simulink model "Senorless"  (R2023a)
settings: Solver=FixedStepDiscrete  StartTime=0.0  StopTime=5  FixedStep=1/FOC_FRQ  RelTol=1e-3
values from neighbouring files (symbols this model uses):
  ADC_REF = 3.6    [Senorless.sldd]
  ADC_SAMPLE_MAX = 32767.0    [Senorless.sldd]
  AMP_GAIN = 16.0    [Senorless.sldd]
  CURR_INPUT = 3276.0    [Senorless.sldd]
  CURR_KI = 380.0    [Senorless.sldd]
  CURR_KP = 0.04    [Senorless.sldd]
  CURR_LIMIT = 0.95    [Senorless.sldd]
  CURR_OVER = 6.0    [Senorless.sldd]
  CURR_POINT_GAIN = 7.0    [Senorless.sldd]
  CURR_STEP = 32760.0    [Senorless.sldd]
  CURR_UNDER = 0.03    [Senorless.sldd]
  CURR_WIDTH = 6552.0    [Senorless.sldd]
  FOC_FRQ = 25000.0    [Senorless.sldd]
  GAMMA = 32767.0    [Senorless.sldd]
  IMAX = 10.0    [Senorless.sldd]
  LPF_FRQ = 2000.0    [Senorless.sldd]
  MOTOR_DAMPER = 2.06E-7    [Senorless.sldd]
  MOTOR_FLUX = 0.00212352    [Senorless.sldd]
  MOTOR_INERTIA = 4.0E-7    [Senorless.sldd]
  MOTOR_LS = 0.000536    [Senorless.sldd]
  MOTOR_PN = 7.0    [Senorless.sldd]
  MOTOR_RS = 4.0    [Senorless.sldd]
  OPEN_IQ = 0.28    [Senorless.sldd]
  OPEN_IQ_MIN = 0.05    [Senorless.sldd]
  OPEN_IQ_SLOW = 0.1    [Senorless.sldd]
  OPEN_SPD = 1000.0    [Senorless.sldd]
  OPEN_SPD_SLOW = 180.0    [Senorless.sldd]
  OPEN_TIME = 0.5    [Senorless.sldd]
  OPEN_TIME_NFO = 0.5    [Senorless.sldd]
  PLL_LIMIT = 0.9    [Senorless.sldd]
  PLL_WIDTH = 800.0    [Senorless.sldd]
  PWM_FRQ = 96000000.0    [Senorless.sldd]
  RS_HUNT = 0.02    [Senorless.sldd]
  SMOK_FRQ = 600.0    [Senorless.sldd]
  SPD_LIMIT = 0.9    [Senorless.sldd]
  SPD_LPF_LEVEL = 0.0    [Senorless.sldd]
  SPD_MAX = 12000.0    [Senorless.sldd]
  SPD_MIN = 4000.0    [Senorless.sldd]
  SPD_REDUCE = 380.0    [Senorless.sldd]
  SPD_STEP = 6.0    [Senorless.sldd]
  SPD_WIDTH = 20.0    [Senorless.sldd]
  THETA_ERR_LIMIT = 8192.0    [Senorless.sldd]
  TS_POINT_GAIN = 10.0    [Senorless.sldd]
  UDC = 48.0    [Senorless.sldd]
  UDC_GAIN = 21.0    [Senorless.sldd]
  UDC_POINT_GAIN = 10.0    [Senorless.sldd]
undefined symbols (not defined in the file or in its folder): curr_q_ki, curr_q_kp, DiscIntNeverNeededParam, magnitude, PLL_LPF_LEVEL, Udc
libraries: simulink x20, slpidlib x5, mcbcontrolslib x2, mcbplantlib x1, autolibpmsmexterior x1, spspowerguiLib x1
(part 7 of 8)

== system Senorless/FOC_PointModel/idq_Controller/PI Controller2/积分器//双边沿初始化 ==
  Ki : Inport
  input : Inport  Port=2
  Xo : Inport  Port=3
  Reset : Inport  Port=4
  Constant : Constant  Value=32767*32767  OutDataTypeStr=int32
  Data Store Memory : DataStoreMemory  DataStoreName=tmp  WriteAfterWriteMsg=warning  ShowAdditionalParam=off  OutDataTypeStr=int32
  Data Store Read : DataStoreRead  DataStoreName=tmp  IndexOptions=Index vector (dialog)  Indices=1  OutputSizes=1
  Data Store Read1 : DataStoreRead  DataStoreName=Ts_Point  IndexOptions=Index vector (dialog)  Indices=1  OutputSizes=1
  Data Store Read3 : DataStoreRead  DataStoreName=Curr_Limit  IndexOptions=Index vector (dialog)  Indices=1  OutputSizes=1
  Data Store Write : DataStoreWrite  DataStoreName=tmp  IndexOptions=Index vector (dialog)  Indices=1  OutputSizes=1
  Data Type Conversion : DataTypeConversion  OutDataTypeStr=int16  SaturateOnIntegerOverflow=off
  Data Type Conversion2 : DataTypeConversion  OutDataTypeStr=int32  SaturateOnIntegerOverflow=off
  Data Type Conversion3 : DataTypeConversion  Commented=on  OutDataTypeStr=int16  SaturateOnIntegerOverflow=off
  Divide : Product  Commented=on  Inputs=*/  OutDataTypeStr=int32  RndMeth=Zero
  Gain : Gain  Gain=-1  OutDataTypeStr=int32  RndMeth=Zero
  Gain1 : Gain  Gain=-1  OutDataTypeStr=int32  RndMeth=Zero
  MATLAB Function : MATLAB Function  TreatAsAtomicUnit=on
  MATLAB Function1 : MATLAB Function  TreatAsAtomicUnit=on
  MATLAB Function2 : MATLAB Function  TreatAsAtomicUnit=on
  Product1 : Product  OutDataTypeStr=int32  RndMeth=Zero
  Product2 : Product  OutDataTypeStr=int32  RndMeth=Zero
  Reset_Block : Subsystem
  Scope : Scope  NumInputPorts=2
  Sum : Sum  Inputs=|++  OutDataTypeStr=int32  RndMeth=Zero
  Sum1 : Sum  Inputs=|+-  OutDataTypeStr=int32  RndMeth=Zero
  Sum2 : Sum  Inputs=-+  OutDataTypeStr=int32  RndMeth=Zero
  Ts适当放大的缩小系数， 详见初始化模块 : ArithShift  Commented=on  BitShiftNumber=TS_POINT_GAIN  DiagnosticForOORShift=Error
  Unit Delay : UnitDelay  SampleTime=-1  HasFrameUpgradeWarning=on
  周期定点化适当放大2^n : Constant  Value=TS_POINT_GAIN
  积分器运行频率 : Constant  Commented=on  Value=FOC_FRQ
  这个是缩小周期增益的 : ArithShift  BitShiftNumber=15  DiagnosticForOORShift=Error
  output : Outport
  wires:
  Data Type Conversion/1 -> Product1/2
  MATLAB Function1/1(out) -> Sum/1, Sum1/2, Scope/2
  [Limit1] -> MATLAB Function1/2(up), Gain1/1
  Gain1/1 -> MATLAB Function1/3(low)
  [limit] -> MATLAB Function/2(up), Gain/1
  Gain/1 -> MATLAB Function/3(low)
  Sum2/1 -> [Limit1]
  Data Store Read3/1 -> [limit], Sum2/1
  Constant/1 -> Sum2/2
  周期定点化适当放大2^n/1 -> MATLAB Function2/2(n)
  input/1 -> Product2/2
  Data Store Read1/1 -> Product2/1
  Sum1/1 -> Reset_Block/1(Xo)
  Data Type Conversion2/1 -> Sum1/1
  Product1/1 -> MATLAB Function1/1(in), Scope/1
  Sum/1 -> MATLAB Function/1(in)
  MATLAB Function2/1(out) -> Product1/1
  Reset/1 -> Reset_Block/Trigger
  Ki/1 -> MATLAB Function2/1(in)
  这个是缩小周期增益的/1 -> Data Type Conversion/1
  Product2/1 -> 这个是缩小周期增益的/1
  Data Type Conversion3/1 -> Divide/2
  Xo/1 -> Data Type Conversion2/1
  积分器运行频率/1 -> Data Type Conversion3/1
  Unit Delay/1 -> Data Store Write/1
  Data Store Read/1 -> Sum/2
  MATLAB Function/1(out) -> Unit Delay/1, output/1

== system Senorless/FOC_PointModel/加速强拖/加速积分角度/积分器 ==
  K_p : Inport
  input : Inport  Port=2
  Xo : Inport  Port=3
  Reset : Inport  Port=4
  Data Store Memory : DataStoreMemory  DataStoreName=tmp  WriteAfterWriteMsg=warning  ShowAdditionalParam=off
  Data Store Read : DataStoreRead  DataStoreName=tmp  IndexOptions=Index vector (dialog)  Indices=1  OutputSizes=1
  Data Store Write : DataStoreWrite  DataStoreName=tmp  IndexOptions=Index vector (dialog)  Indices=1  OutputSizes=1
  Data Type Conversion2 : DataTypeConversion  OutDataTypeStr=int32  SaturateOnIntegerOverflow=off
  Data Type Conversion3 : DataTypeConversion  OutDataTypeStr=int32  SaturateOnIntegerOverflow=off
  Divide : Product  Inputs=*/  OutDataTypeStr=int32  RndMeth=Zero
  Product : Product  OutDataTypeStr=int64  RndMeth=Zero
  Product1 : Product  OutDataTypeStr=int64  RndMeth=Zero
  Reset_Block : Subsystem
  Sum : Sum  Inputs=|++  OutDataTypeStr=int64  RndMeth=Zero
  Unit Delay : UnitDelay  SampleTime=-1  HasFrameUpgradeWarning=on
  积分器运行频率 : Constant  Value=FOC_FRQ
  output : Outport
  wires:
  K_p/1 -> Product1/1, Product/2
  Reset/1 -> Reset_Block/Trigger
  Data Store Read/1 -> Sum/2
  Unit Delay/1 -> Data Store Write/1
  Product/1 -> Reset_Block/1(Xo)
  Divide/1 -> Product1/2
  input/1 -> Divide/1
  Product1/1 -> Sum/1
  积分器运行频率/1 -> Data Type Conversion3/1
  Data Type Conversion3/1 -> Divide/2
  Xo/1 -> Data Type Conversion2/1
  Data Type Conversion2/1 -> Product/1
  Sum/1 -> Unit Delay/1, output/1

== system Senorless/FOC_PointModel/加速强拖/加速积分角度/积分器2 ==
  note: 此处相减作用是与后面的++相抵消，这样初始化后第一个输出值就是reset值，不然是reset值+Kp*input值
  K_p : Inport
  input : Inport  Port=2
  Xo : Inport  Port=3
  Reset : Inport  Port=4
  Data Store Memory : DataStoreMemory  DataStoreName=tmp  WriteAfterWriteMsg=warning  ShowAdditionalParam=off
  Data Store Read : DataStoreRead  DataStoreName=tmp  IndexOptions=Index vector (dialog)  Indices=1  OutputSizes=1
  Data Store Write : DataStoreWrite  DataStoreName=tmp  IndexOptions=Index vector (dialog)  Indices=1  OutputSizes=1
  Data Type Conversion2 : DataTypeConversion  OutDataTypeStr=int32  SaturateOnIntegerOverflow=off
  Data Type Conversion3 : DataTypeConversion  OutDataTypeStr=int32  SaturateOnIntegerOverflow=off
  Divide : Product  Inputs=*/  OutDataTypeStr=int32  RndMeth=Zero
  Product : Product  OutDataTypeStr=int64  RndMeth=Zero
  Product1 : Product  OutDataTypeStr=int64  RndMeth=Zero
  Reset_Block : Subsystem
  Sum : Sum  Inputs=|++  OutDataTypeStr=int64  RndMeth=Zero
  Sum1 : Sum  Inputs=|+-  OutDataTypeStr=int64  RndMeth=Zero
  Unit Delay : UnitDelay  SampleTime=-1  HasFrameUpgradeWarning=on
  积分器运行频率 : Constant  Value=FOC_FRQ
  output : Outport
  wires:
  K_p/1 -> Product1/1, Product/2
  Reset/1 -> Reset_Block/Trigger
  Data Store Read/1 -> Sum/2
  Sum/1 -> Unit Delay/1, output/1
  Unit Delay/1 -> Data Store Write/1
  Product/1 -> Sum1/1
  Divide/1 -> Product1/2
  input/1 -> Divide/1
  Product1/1 -> Sum1/2, Sum/1
  积分器运行频率/1 -> Data Type Conversion3/1
  Data Type Conversion3/1 -> Divide/2
  Xo/1 -> Data Type Conversion2/1
  Data Type Conversion2/1 -> Product/1
  Sum1/1 -> Reset_Block/1(Xo)

== system Senorless/FOC_PointModel/加速强拖/加速积分角度/积分器3 ==
  input : Inport
  Constant : Constant  OutDataTypeStr=int16
  Data Store Read1 : DataStoreRead  DataStoreName=Ts_Point  IndexOptions=Index vector (dialog)  Indices=1  OutputSizes=1
  Product1 : Product  OutDataTypeStr=int32  RndMeth=Zero
  Product2 : Product  OutDataTypeStr=int32  RndMeth=Zero
  Shift Arithmetic : ArithShift  BitShiftNumberSource=Input port  BitShiftNumber=8  BitShiftDirection=Right
      settings: InputPortMap=u0,p1
  Sum : Sum  Inputs=++|  OutDataTypeStr=int32  RndMeth=Zero
  Unit Delay : UnitDelay  SampleTime=-1  HasFrameUpgradeWarning=on
  周期定点化适当放大2^n : Constant  Value=TS_POINT_GAIN
  这个是缩小周期增益的 : ArithShift  BitShiftNumber=15  DiagnosticForOORShift=Error
  output : Outport
  wires:
  周期定点化适当放大2^n/1 -> Shift Arithmetic/2
  Shift Arithmetic/1 -> Product2/2
  Data Store Read1/1 -> Product2/1
  input/1 -> Shift Arithmetic/1
  Product2/1 -> 这个是缩小周期增益的/1
  Sum/1 -> Unit Delay/1, output/1
  这个是缩小周期增益的/1 -> Product1/1
  Constant/1 -> Product1/2
  Product1/1 -> Sum/2
  Unit Delay/1 -> Sum/1

== system Senorless/FOC_PointModel/加速强拖/加速积分角度/积分器4 ==
  input : Inport
  Constant : Constant  OutDataTypeStr=int16
  Data Store Read1 : DataStoreRead  DataStoreName=Ts_Point  IndexOptions=Index vector (dialog)  Indices=1  OutputSizes=1
  Product1 : Product  OutDataTypeStr=int32  RndMeth=Zero
  Product2 : Product  OutDataTypeStr=int32  RndMeth=Zero
  Shift Arithmetic : ArithShift  BitShiftNumberSource=Input port  BitShiftNumber=8  BitShiftDirection=Right
      settings: InputPortMap=u0,p1
  Sum : Sum  Inputs=++|  OutDataTypeStr=int32  RndMeth=Zero
  Unit Delay : UnitDelay  SampleTime=-1  HasFrameUpgradeWarning=on
  周期定点化适当放大2^n : Constant  Value=TS_POINT_GAIN
  这个是缩小周期增益的 : ArithShift  BitShiftNumber=15  DiagnosticForOORShift=Error
  output : Outport
  wires:
  Unit Delay/1 -> Sum/1
  Product1/1 -> Sum/2
  Constant/1 -> Product1/2
  这个是缩小周期增益的/1 -> Product1/1
  Sum/1 -> output/1, Unit Delay/1
  Product2/1 -> 这个是缩小周期增益的/1
  input/1 -> Shift Arithmetic/1
  Data Store Read1/1 -> Product2/1
  Shift Arithmetic/1 -> Product2/2
  周期定点化适当放大2^n/1 -> Shift Arithmetic/2

== system Senorless/FOC_PointModel/观测器闭环//速度环/PI Controller/积分器 ==
  Ki : Inport
  input : Inport  Port=2
  Constant : Constant  Value=32767  OutDataTypeStr=int32
  Data Store Read1 : DataStoreRead  DataStoreName=Ts_Point  IndexOptions=Index vector (dialog)  Indices=1  OutputSizes=1
  Data Store Read3 : DataStoreRead  DataStoreName=Speed_Limit  IndexOptions=Index vector (dialog)  Indices=1  OutputSizes=1
  Data Type Conversion1 : DataTypeConversion  OutDataTypeStr=int16  SaturateOnIntegerOverflow=off
  Gain1 : Gain  Gain=-1  OutDataTypeStr=int32  RndMeth=Zero
  Gain2 : Gain  Gain=-1  OutDataTypeStr=int32  RndMeth=Zero
  MATLAB Function : MATLAB Function  TreatAsAtomicUnit=on
  MATLAB Function1 : MATLAB Function  TreatAsAtomicUnit=on
  Product1 : Product  OutDataTypeStr=int32  RndMeth=Zero
  Product2 : Product  OutDataTypeStr=int32  RndMeth=Zero
  Scope : Scope  NumInputPorts=2
  Shift Arithmetic : ArithShift  BitShiftNumberSource=Input port  BitShiftNumber=8  BitShiftDirection=Right
      settings: InputPortMap=u0,p1
  Sum : Sum  Inputs=|++  OutDataTypeStr=int32  RndMeth=Zero
  Sum2 : Sum  Inputs=-+  OutDataTypeStr=int32  RndMeth=Zero
  Unit Delay : UnitDelay  SampleTime=-1  HasFrameUpgradeWarning=on
  周期定点化适当放大2^n : Constant  Value=TS_POINT_GAIN
  这个是缩小周期增益的 : ArithShift  BitShiftNumber=15  DiagnosticForOORShift=Warning
  output : Outport
  wires:
  Constant/1 -> Sum2/2
  Sum2/1 -> [Limit1]
  [limit] -> Gain2/1, MATLAB Function/2(up)
  Gain1/1 -> MATLAB Function1/3(low)
  [Limit1] -> Gain1/1, MATLAB Function1/2(up)
  MATLAB Function1/1(out) -> Sum/1
  Sum/1 -> MATLAB Function/1(in)
  Ki/1 -> Product1/1
  Product2/1 -> Shift Arithmetic/1
  Data Store Read1/1 -> Product2/1
  周期定点化适当放大2^n/1 -> Shift Arithmetic/2
  MATLAB Function/1(out) -> Unit Delay/1, output/1
  input/1 -> Product2/2
  Product1/1 -> 这个是缩小周期增益的/1
  这个是缩小周期增益的/1 -> MATLAB Function1/1(in)
  Data Store Read3/1 -> Sum2/1, [limit]
  Data Type Conversion1/1 -> Scope/1, Product1/2
  Gain2/1 -> MATLAB Function/3(low)
  Shift Arithmetic/1 -> Scope/2, Data Type Conversion1/1
  Unit Delay/1 -> Sum/2

== system Senorless/FOC_PointModel/观测器闭环//速度环/积分器//上升沿初始化/Reset_Block ==
  Xo : Inport
  Trigger : TriggerPort  VariantControl=(inherit)  OutputDataType=int8  InitialTriggerSignalState=zero  PortDimensions=1
  Data Store Write1 : DataStoreWrite  DataStoreName=tmp  IndexOptions=Index vector (dialog)  Indices=1  OutputSizes=1
  wires:
  Xo/1 -> Data Store Write1/1

== system Senorless/FOC_PointModel/Observers/PLL/PI Controller/积分器 ==
  Ki : Inport
  input : Inport  Port=2
  Constant : Constant  Value=32767*32767  OutDataTypeStr=int32
  Data Store Read1 : DataStoreRead  DataStoreName=Ts_Point  IndexOptions=Index vector (dialog)  Indices=1  OutputSizes=1
  Data Store Read3 : DataStoreRead  DataStoreName=PLL_Limit  IndexOptions=Index vector (dialog)  Indices=1  OutputSizes=1
  Data Type Conversion3 : DataTypeConversion  Commented=on  OutDataTypeStr=int16  SaturateOnIntegerOverflow=off
  Divide : Product  Commented=on  Inputs=*/  OutDataTypeStr=int32  RndMeth=Zero
  Gain : Gain  Gain=-1  OutDataTypeStr=int32  RndMeth=Zero
  Product1 : Product  OutDataTypeStr=int32  RndMeth=Zero
  Product2 : Product  OutDataTypeStr=int32  RndMeth=Zero
  Saturation Dynamic2 : simulink/Discontinuities/Saturation Dynamic  OutMin=[]  OutMax=[]  OutDataTypeStr=Inherit: Same as second input  OutDataType=fixdt(1, 16)  OutScaling=2^-10  RndMeth=Zero  DoSatur=off
  Shift Arithmetic : ArithShift  BitShiftNumberSource=Input port  BitShiftNumber=8  BitShiftDirection=Right
      settings: InputPortMap=u0,p1
  Sum : Sum  Inputs=|++  OutDataTypeStr=int32  RndMeth=Zero
  Sum2 : Sum  Inputs=-+  OutDataTypeStr=int32  RndMeth=Zero
  Ts适当放大的缩小系数， 详见初始化模块 : ArithShift  Commented=on  BitShiftNumber=TS_POINT_GAIN  DiagnosticForOORShift=Error
  Unit Delay : UnitDelay  SampleTime=-1  HasFrameUpgradeWarning=on
  周期定点化适当放大2^n : Constant  Value=TS_POINT_GAIN
  积分器运行频率 : Constant  Commented=on  Value=FOC_FRQ
  这个是缩小周期增益的 : ArithShift  BitShiftNumber=15  DiagnosticForOORShift=Error
  output : Outport
  wires:
  积分器运行频率/1 -> Data Type Conversion3/1
  Data Type Conversion3/1 -> Divide/2
  Product2/1 -> 这个是缩小周期增益的/1
  Ki/1 -> Shift Arithmetic/1
  Shift Arithmetic/1 -> Product1/1
  Data Store Read1/1 -> Product2/1
  input/1 -> Product2/2
  周期定点化适当放大2^n/1 -> Shift Arithmetic/2
  [Limit] -> Gain/1
  Data Store Read3/1 -> Sum2/1, [Limit]
  Constant/1 -> Sum2/2
  Sum2/1 -> [Limit1]
  这个是缩小周期增益的/1 -> Product1/2
  Unit Delay/1 -> Sum/2
  Gain/1 -> Saturation Dynamic2/3
  Sum/1 -> Saturation Dynamic2/2
  [Limit] -> Saturation Dynamic2/1
  Saturation Dynamic2/1 -> Unit Delay/1, output/1
  Product1/1 -> Sum/1

== system Senorless/FOC_PointModel/Observers/PLL2/PI Controller/积分器 ==
  Ki : Inport
  input : Inport  Port=2
  Constant : Constant  Value=32767*32767  OutDataTypeStr=int32
  Data Store Read1 : DataStoreRead  DataStoreName=Ts_Point  IndexOptions=Index vector (dialog)  Indices=1  OutputSizes=1
  Data Store Read3 : DataStoreRead  DataStoreName=PLL_Limit  IndexOptions=Index vector (dialog)  Indices=1  OutputSizes=1
  Data Type Conversion3 : DataTypeConversion  Commented=on  OutDataTypeStr=int16  SaturateOnIntegerOverflow=off
  Divide : Product  Commented=on  Inputs=*/  OutDataTypeStr=int32  RndMeth=Zero
  Gain : Gain  Gain=-1  OutDataTypeStr=int32  RndMeth=Zero
  Product1 : Product  OutDataTypeStr=int32  RndMeth=Zero
  Product2 : Product  OutDataTypeStr=int32  RndMeth=Zero
  Saturation Dynamic2 : simulink/Discontinuities/Saturation Dynamic  OutMin=[]  OutMax=[]  OutDataTypeStr=Inherit: Same as second input  OutDataType=fixdt(1, 16)  OutScaling=2^-10  RndMeth=Zero  DoSatur=off
  Shift Arithmetic : ArithShift  BitShiftNumberSource=Input port  BitShiftNumber=8  BitShiftDirection=Right
      settings: InputPortMap=u0,p1
  Sum : Sum  Inputs=|++  OutDataTypeStr=int32  RndMeth=Zero
  Sum2 : Sum  Inputs=-+  OutDataTypeStr=int32  RndMeth=Zero
  Ts适当放大的缩小系数， 详见初始化模块 : ArithShift  Commented=on  BitShiftNumber=TS_POINT_GAIN  DiagnosticForOORShift=Error
  Unit Delay : UnitDelay  SampleTime=-1  HasFrameUpgradeWarning=on
  周期定点化适当放大2^n : Constant  Value=TS_POINT_GAIN
  积分器运行频率 : Constant  Commented=on  Value=FOC_FRQ
  这个是缩小周期增益的 : ArithShift  BitShiftNumber=15  DiagnosticForOORShift=Error
  output : Outport
  wires:
  Product1/1 -> Sum/1
  Saturation Dynamic2/1 -> output/1, Unit Delay/1
  [Limit] -> Saturation Dynamic2/1
  Sum/1 -> Saturation Dynamic2/2
  Gain/1 -> Saturation Dynamic2/3
  Unit Delay/1 -> Sum/2
  这个是缩小周期增益的/1 -> Product1/2
  Sum2/1 -> [Limit1]
  Constant/1 -> Sum2/2
  Data Store Read3/1 -> [Limit], Sum2/1
  [Limit] -> Gain/1
  周期定点化适当放大2^n/1 -> Shift Arithmetic/2
  input/1 -> Product2/2
  Data Store Read1/1 -> Product2/1
  Shift Arithmetic/1 -> Product1/1
  Ki/1 -> Shift Arithmetic/1
  Product2/1 -> 这个是缩小周期增益的/1
  Data Type Conversion3/1 -> Divide/2
  积分器运行频率/1 -> Data Type Conversion3/1

== system Senorless/FOC_PointModel/idq_Controller/PI Controller2/积分器//双边沿初始化/Reset_Block ==
  Xo : Inport
  Trigger : TriggerPort  TriggerType=either  VariantControl=(inherit)  OutputDataType=int8  InitialTriggerSignalState=zero  PortDimensions=1
  Data Store Write1 : DataStoreWrite  DataStoreName=tmp  IndexOptions=Index vector (dialog)  Indices=1  OutputSizes=1
  wires:
  Xo/1 -> Data Store Write1/1

== system Senorless/FOC_PointModel/加速强拖/加速积分角度/积分器/Reset_Block ==
  Xo : Inport
  Trigger : TriggerPort  VariantControl=(inherit)  OutputDataType=int8  InitialTriggerSignalState=zero  PortDimensions=1
  Data Store Write1 : DataStoreWrite  DataStoreName=tmp  IndexOptions=Index vector (dialog)  Indices=1  OutputSizes=1
  wires:
  Xo/1 -> Data Store Write1/1

== system Senorless/FOC_PointModel/加速强拖/加速积分角度/积分器2/Reset_Block ==
  Xo : Inport
  Trigger : TriggerPort  VariantControl=(inherit)  OutputDataType=int8  InitialTriggerSignalState=zero  PortDimensions=1
  Data Store Write1 : DataStoreWrite  DataStoreName=tmp  IndexOptions=Index vector (dialog)  Indices=1  OutputSizes=1
  wires:
  Xo/1 -> Data Store Write1/1

== stateflow chart Senorless/FOC_PointModel/Chart ==
  state StopStage%出错暂停
    en:
    du:
    Reset = 1;
    ex:
  state IDLE
    en:
    du:
    Motor_State = 0;
    Reset = 0;
    ex:
  state SlowOpen%缓慢强拖
    en:
    du:
    Motor_State = 5;
    Reset = 0;
    ex:
  state AlignStage%对齐
    en:
    du:
    Motor_State = 1;
    ex:
  state OpenStage%降力矩
    en:
    Over_Curr_Cnt = 0;
    du:
    Motor_State = 3;
    ex:
  state SpeedupStage%加速
    en:
    du:
    Motor_State = 2;
    ex:
  state RunStage%闭环
    en:
    du:
    Motor_State = 4;
    ex:
  state EndStage%出错结束
    en:
    du:
    Reset = 1;
    ex:
  StopStage%出错暂停 -> IDLE : [after(200,msec)]
  AlignStage%对齐 -> StopStage%出错暂停 [order 3] : [OverCurr_Err == 1]
  SpeedupStage%加速 -> StopStage%出错暂停 [order 3] : [OverCurr_Err == 1]
  OpenStage%降力矩 -> StopStage%出错暂停 [order 3] : [OverCurr_Err == 1]
  OpenStage%降力矩 -> StopStage%出错暂停 [order 4] : [after(500,msec)]
  (default) -> IDLE
  IDLE -> SlowOpen%缓慢强拖 [order 2] : [Slow_OnOff == 1 && after(10,msec)]
  AlignStage%对齐 -> SpeedupStage%加速 [order 1] : [after(10,msec)]
  SpeedupStage%加速 -> OpenStage%降力矩 [order 2] : [after(OPEN_TIME,sec) ]
  IDLE -> AlignStage%对齐 [order 1] : [Motor_OnOff ==1 && after(10,msec)]
  OpenStage%降力矩 -> RunStage%闭环 [order 2] : [after(250,msec)&&Theta_Err<THETA_ERR_LIMIT]
  RunStage%闭环 -> EndStage%出错结束 [order 2] : [Run_Err == 1]
  SlowOpen%缓慢强拖 -> IDLE : [Slow_OnOff == 0]
  EndStage%出错结束 -> IDLE : [Motor_OnOff ==0]
  RunStage%闭环 -> IDLE [order 1] : [Motor_OnOff ==0]
  SpeedupStage%加速 -> IDLE [order 1] : [Motor_OnOff ==0]
  AlignStage%对齐 -> IDLE [order 2] : [Motor_OnOff == 0]
  OpenStage%降力矩 -> IDLE [order 1] : [Motor_OnOff ==0]
  data: Motor_OnOff input int16; Slow_OnOff input int16; OPEN_TIME parameter single; Theta_Err input int32; THETA_ERR_LIMIT parameter int16; Reset output int16; Run_Err input boolean; OverCurr_Err input boolean; Over_Curr_Cnt local uint8 =0; Motor_State output uint8

== matlab function Senorless/FOC_PointModel/Sin_512 ==
  data: angle_i16 input; sin_val output; cos_val output
function [sin_val, cos_val] = trig512_lookup_int16(angle_i16)
% trig512_lookup_int16 - 使用512点正弦表实现 sin 和 cos 查表（纯整数运算）
%
% 输入:
%   angle_i16 - int16 类型，范围 [-32768, 32767]
%              表示 -π ~ π（或 -180° ~ 179.9°）
% 输出:
%   sin_val   - int16 类型，正弦值范围 [-32768, 32767]
%   cos_val   - int16 类型，余弦值范围 [-32768, 32767]

    %#codegen

    % 获取正弦表（int16 类型，512 点）
    coder.const('get_sine_table_512pt');
    persistent sin512;
    if isempty(sin512)
        sin512 = get_sine_table_512pt();  % 返回 int16 类型的 512 点表
    end

    % 计算索引：将 [-32768, 32767] 映射到 [0, 511]
    index = bitand(bitshift(angle_i16, -7), 511);  % 右移 7 位并取模 512

    % 获取 sin 值（MATLAB 表从 1 开始）
    sin_val = int16(sin512(index + 1));

    % 获取 cos 值: cos(x) = sin(x + 90°) = sin(x + 128 in 512点表)
    cos_index = bitand(int32(index) + 128, 511);  % 快速取模
    cos_val = int16(sin512(cos_index + 1));
end

% =============================
% 512点正弦表定义（int16类型）
% =============================
function sin_table = get_sine_table_512pt()
    sin_table = int16([
 0 ,   402 ,   804 ,  1207 ,  1609 , ...
      2011 ,  2412 ,  2814 ,  3214 ,  3615 , ...
      4015 ,  4414 ,  4812 ,  5210 ,  5607 , ...
      6003 ,  6398 ,  6793 ,  7186 ,  7578 , ...
      7969 ,  8359 ,  8747 ,  9135 ,  9521 , ...
      9905 , 10288 , 10669 , 11049 , 11427 , ...
     11804 , 12178 , 12551 , 12922 , 13291 , ...
     13658 , 14022 , 14385 , 14746 , 15104 , ...
     15460 , 15814 , 16165 , 16514 , 16860 , ...
     17204 , 17546 , 17884 , 18220 , 18553 , ...
     18884 , 19211 , 19536 , 19857 , 20176 , ...
     20492 , 20804 , 21114 , 21420 , 21723 , ...
     22023 , 22319 , 22612 , 22902 , 23188 , ...
     23470 , 23750 , 24025 , 24297 , 24565 , ...
     24830 , 25090 , 25347 , 25601 , 25850 , ...
     26095 , 26337 , 26574 , 26808 , 27037 , ...
     27263 , 27484 , 27701 , 27914 , 28123 , ...
     28327 , 28527 , 28723 , 28915 , 29102 , ...
     29285 , 29463 , 29637 , 29806 , 29971 , ...
     30132 , 30288 , 30439 , 30586 , 30728 , ...
     30865 , 30998 , 31126 , 31250 , 31368 , ...
     31482 , 31592 , 31696 , 31796 , 31891 , ...
     31981 , 32066 , 32146 , 32222 , 32293 , ...
     32359 , 32419 , 32476 , 32527 , 32573 , ...
     32614 , 32651 , 32682 , 32709 , 32730 , ...
     32747 , 32759 , 32766 , 32767 , 32764 , ...
     32756 , 32743 , 32725 , 32703 , 32675 , ...
     32642 , 32604 , 32562 , 32514 , 32462 , ...
     32405 , 32343 , 32275 , 32204 , 32127 , ...
     32045 , 31959 , 31867 , 31771 , 31670 , ...
     31565 , 31454 , 31339 , 31219 , 31095 , ...
     30965 , 30831 , 30693 , 30549 , 30402 , ...
     30249 , 30092 , 29930 , 29764 , 29594 , ...
     29419 , 29239 , 29055 , 28867 , 28674 , ...
     28478 , 28276 , 28071 , 27861 , 27647 , ...
     27429 , 27207 , 26980 , 26750 , 26515 , ...
     26277 , 26034 , 25788 , 25538 , 25284 , ...
     25026 , 24764 , 24498 , 24229 , 23956 , ...
     23680 , 23400 , 23117 , 22830 , 22539 , ...
     22245 , 21948 , 21647 , 21344 , 21037 , ...
     20726 , 20413 , 20097 , 19777 , 19455 , ...
     19130 , 18801 , 18470 , 18136 , 17800 , ...
     17461 , 17119 , 16774 , 16427 , 16078 , ...
     15726 , 15371 , 15015 , 14656 , 14295 , ...
     13931 , 13566 , 13199 , 12829 , 12458 , ...
     12085 , 11710 , 11333 , 10954 , 10574 , ...
     10192 ,  9809 ,  9424 ,  9038 ,  8650 , ...
      8262 ,  7871 ,  7480 ,  7088 ,  6694 , ...
      6300 ,  5904 ,  5508 ,  5111 ,  4713 , ...
      4314 ,  3915 ,  3515 ,  3114 ,  2713 , ...
      2312 ,  1910 ,  1508 ,  1106 ,   704 , ...
       301 ,  -100 ,  -503 ,  -905 , -1307 , ...
     -1709 , -2111 , -2513 , -2914 , -3315 , ...
     -3715 , -4114 , -4513 , -4912 , -5309 , ...
     -5706 , -6102 , -6497 , -6891 , -7284 , ...
     -7676 , -8067 , -8456 , -8844 , -9231 , ...
     -9617 ,-10001 ,-10383 ,-10764 ,-11144 , ...
    -11521 ,-11897 ,-12271 ,-12644 ,-13014 , ...
    -13383 ,-13749 ,-14113 ,-14475 ,-14835 , ...
    -15193 ,-15549 ,-15902 ,-16253 ,-16601 , ...
    -16947 ,-17290 ,-17630 ,-17968 ,-18304 , ...
    -18636 ,-18966 ,-19293 ,-19616 ,-19937 , ...
    -20255 ,-20570 ,-20882 ,-21191 ,-21496 , ...
    -21798 ,-22097 ,-22393 ,-22685 ,-22973 , ...
    -23259 ,-23541 ,-23819 ,-24093 ,-24364 , ...
    -24632 ,-24895 ,-25155 ,-25411 ,-25663 , ...
    -25912 ,-26156 ,-26397 ,-26633 ,-26866 , ...
    -27094 ,-27318 ,-27538 ,-27755 ,-27966 , ...
    -28174 ,-28377 ,-28577 ,-28771 ,-28962 , ...
    -29148 ,-29330 ,-29507 ,-29680 ,-29848 , ...
    -30012 ,-30171 ,-30326 ,-30476 ,-30622 , ...
    -30763 ,-30899 ,-31031 ,-31157 ,-31280 , ...
    -31397 ,-31510 ,-31618 ,-31721 ,-31820 , ...
    -31914 ,-32003 ,-32087 ,-32166 ,-32240 , ...
    -32310 ,-32374 ,-32434 ,-32489 ,-32539 , ...
    -32584 ,-32624 ,-32659 ,-32689 ,-32715 , ...
    -32735 ,-32750 ,-32761 ,-32767 ,-32767 , ...
    -32763 ,-32754 ,-32739 ,-32720 ,-32696 , ...
    -32667 ,-32633 ,-32594 ,-32550 ,-32502 , ...
    -32448 ,-32390 ,-32326 ,-32258 ,-32185 , ...
    -32107 ,-32024 ,-31936 ,-31844 ,-31747 , ...
    -31644 ,-31538 ,-31426 ,-31310 ,-31189 , ...
    -31063 ,-30932 ,-30797 ,-30657 ,-30513 , ...
    -30364 ,-30210 ,-30052 ,-29889 ,-29722 , ...
    -29550 ,-29374 ,-29194 ,-29009 ,-28819 , ...
    -28626 ,-28428 ,-28225 ,-28019 ,-27808 , ...
    -27593 ,-27374 ,-27150 ,-26923 ,-26692 , ...
    -26456 ,-26217 ,-25973 ,-25726 ,-25475 , ...
    -25219 ,-24961 ,-24698 ,-24432 ,-24161 , ...
    -23888 ,-23610 ,-23330 ,-23045 ,-22757 , ...
    -22466 ,-22171 ,-21873 ,-21572 ,-21267 , ...
    -20959 ,-20648 ,-20334 ,-20017 ,-19697 , ...
    -19374 ,-19048 ,-18719 ,-18387 ,-18052 , ...
    -17715 ,-17375 ,-17033 ,-16688 ,-16340 , ...
    -15990 ,-15637 ,-15282 ,-14925 ,-14566 , ...
    -14204 ,-13840 ,-13474 ,-13106 ,-12737 , ...
    -12365 ,-11991 ,-11616 ,-11238 ,-10859 , ...
    -10479 ,-10097 , -9713 , -9328 , -8941 , ...
     -8553 , -8164 , -7774 , -7382 , -6989 , ...
     -6596 , -6201 , -5805 , -5409 , -5011 , ...
     -4613 , -4214 , -3815 , -3415 , -3014 , ...
     -2613 , -2212 , -1810 , -1408 , -1006 , ...
      -603 ,  -201 ...
    ]);
end

== matlab function Senorless/FOC_PointModel/恒速降力矩强拖/FreqGenerator_point2/MATLAB Function1 ==
  data: u input; y output; K_fixed input; freq_kHz input; resetTrig input; resetValue input; lowerLimit input; upperLimit input
function y = edgeTri_fixedPointIntegrator(u, K_fixed, freq_kHz, resetTrig, resetValue, lowerLimit, upperLimit)
% fixedPointIntegrator - 定点积分器（频率输入 + 复位 + 限幅 + 初始值）
%
% 输入参数说明：
%   u           - 当前输入信号（int32）
%   K_fixed     - 积分增益（已放大后的定点值，int32）
%   freq_kHz    - 控制频率（单位：kHz，如 20 表示 20kHz）
%   resetTrig   - 复位触发信号（uint8，边沿触发复位）
%   resetValue  - 复位时的初始值（int64）
%   lowerLimit  - 输出最小值（int64）
%   upperLimit  - 输出最大值（int64）
%
% 输出：
%   y           - 当前积分输出（int64）

    % 用于检测上升沿
    persistent lastResetState;
    if isempty(lastResetState)
        lastResetState = uint8(1);
    end

    % 状态变量
    persistent integratorState;
    if isempty(integratorState)
        integratorState = int64(0);
    end

    % 检测是否发生边沿触发（上升沿 或 下降沿）
    edgeTriggered = (resetTrig ~= lastResetState);

    % 如果有边沿，则复位积分器
    if edgeTriggered
        integratorState = resetValue;
    else
        % 计算 Ts（单位：μs），即 Ts = 1_000_000 / (freq_kHz * 1000)
        Ts_us = int32(1000 / freq_kHz);  % 精确到 μs（微秒）

        % 计算积分增量：delta = (K_fixed * u * Ts_us) / 1_000_000
        delta = (int64(K_fixed) * int64(u) * int64(Ts_us)) / 1000000;

        % 更新积分状态
        integratorState = integratorState + delta;

        % 饱和处理
        if integratorState > upperLimit
            integratorState = upperLimit;
        elseif integratorState < lowerLimit
            integratorState = lowerLimit;
        end
    end

    % 更新复位信号历史状态
    lastResetState = resetTrig;

    % 输出当前积分结果
    y = integratorState;
end

== matlab function Senorless/FOC_PointModel/恒速降力矩强拖/MATLAB Function ==
  data: u1 input; y output; u2 input; u3 input
function y = fcn(u1,u2,u3)

y = u1;
if u3==0
    y = u2;
end

== matlab function Senorless/FOC_PointModel/Sin2_512 ==
  data: angle_u16 input; sin_val output; cos_val output
function [sin_val, cos_val] = trig512_lookup(angle_u16)
    % trig512_lookup - 使用512点正弦表实现 sin 和 cos 查表（纯整数运算）
    % 输入: angle_u16 - uint16 类型，范围 [0, 65535]
    % 输出: sin_val, cos_val - int16 类型，范围 [-32768, 32767]

    %#codegen

    coder.const('sin_table512');
    % 512点正弦表 (int16)
    persistent sin512;
    if isempty(sin512)
        sin512 = get_sine_table_512pt();  % 假设这个函数返回 int16 类型的 512 点表
    end

    % 计算索引：右移 7 位相当于除以 128（因为 2^7 = 128）
    index = uint16(bitshift(angle_u16, -7));  % 右移 7 位 => index in [0, 511]
    
    % 获取 sin 值
    sin_val = int16(sin512(index + 1));  % MATLAB 表从 1 开始

    % 获取 cos 值: cos(x) = sin(x + 90°) = sin(x + 128 in 512点表)
    cos_index = uint16(mod(uint32(index) + 128, 512));  % 快速取模
    cos_val = int16(sin512(cos_index + 1));  % MATLAB 表从 1 开始
end

% =============================
% 512点正弦表定义（int16类型）
% =============================
function sin_table = get_sine_table_512pt()
    sin_table = int16([
 0 ,   402 ,   804 ,  1207 ,  1609 , ...
      2011 ,  2412 ,  2814 ,  3214 ,  3615 , ...
      4015 ,  4414 ,  4812 ,  5210 ,  5607 , ...
      6003 ,  6398 ,  6793 ,  7186 ,  7578 , ...
      7969 ,  8359 ,  8747 ,  9135 ,  9521 , ...
      9905 , 10288 , 10669 , 11049 , 11427 , ...
     11804 , 12178 , 12551 , 12922 , 13291 , ...
     13658 , 14022 , 14385 , 14746 , 15104 , ...
     15460 , 15814 , 16165 , 16514 , 16860 , ...
     17204 , 17546 , 17884 , 18220 , 18553 , ...
     18884 , 19211 , 19536 , 19857 , 20176 , ...
     20492 , 20804 , 21114 , 21420 , 21723 , ...
     22023 , 22319 , 22612 , 22902 , 23188 , ...
     23470 , 23750 , 24025 , 24297 , 24565 , ...
     24830 , 25090 , 25347 , 25601 , 25850 , ...
     26095 , 26337 , 26574 , 26808 , 27037 , ...
     27263 , 27484 , 27701 , 27914 , 28123 , ...
     28327 , 28527 , 28723 , 28915 , 29102 , ...
     29285 , 29463 , 29637 , 29806 , 29971 , ...
     30132 , 30288 , 30439 , 30586 , 30728 , ...
     30865 , 30998 , 31126 , 31250 , 31368 , ...
     31482 , 31592 , 31696 , 31796 , 31891 , ...
     31981 , 32066 , 32146 , 32222 , 32293 , ...
     32359 , 32419 , 32476 , 32527 , 32573 , ...
     32614 , 32651 , 32682 , 32709 , 32730 , ...
     32747 , 32759 , 32766 , 32767 , 32764 , ...
     32756 , 32743 , 32725 , 32703 , 32675 , ...
     32642 , 32604 , 32562 , 32514 , 32462 , ...
     32405 , 32343 , 32275 , 32204 , 32127 , ...
     32045 , 31959 , 31867 , 31771 , 31670 , ...
     31565 , 31454 , 31339 , 31219 , 31095 , ...
     30965 , 30831 , 30693 , 30549 , 30402 , ...
     30249 , 30092 , 29930 , 29764 , 29594 , ...
     29419 , 29239 , 29055 , 28867 , 28674 , ...
     28478 , 28276 , 28071 , 27861 , 27647 , ...
     27429 , 27207 , 26980 , 26750 , 26515 , ...
     26277 , 26034 , 25788 , 25538 , 25284 , ...
     25026 , 24764 , 24498 , 24229 , 23956 , ...
     23680 , 23400 , 23117 , 22830 , 22539 , ...
     22245 , 21948 , 21647 , 21344 , 21037 , ...
     20726 , 20413 , 20097 , 19777 , 19455 , ...
     19130 , 18801 , 18470 , 18136 , 17800 , ...
     17461 , 17119 , 16774 , 16427 , 16078 , ...
     15726 , 15371 , 15015 , 14656 , 14295 , ...
     13931 , 13566 , 13199 , 12829 , 12458 , ...
     12085 , 11710 , 11333 , 10954 , 10574 , ...
     10192 ,  9809 ,  9424 ,  9038 ,  8650 , ...
      8262 ,  7871 ,  7480 ,  7088 ,  6694 , ...
      6300 ,  5904 ,  5508 ,  5111 ,  4713 , ...
      4314 ,  3915 ,  3515 ,  3114 ,  2713 , ...
      2312 ,  1910 ,  1508 ,  1106 ,   704 , ...
       301 ,  -100 ,  -503 ,  -905 , -1307 , ...
     -1709 , -2111 , -2513 , -2914 , -3315 , ...
     -3715 , -4114 , -4513 , -4912 , -5309 , ...
     -5706 , -6102 , -6497 , -6891 , -7284 , ...
     -7676 , -8067 , -8456 , -8844 , -9231 , ...
     -9617 ,-10001 ,-10383 ,-10764 ,-11144 , ...
    -11521 ,-11897 ,-12271 ,-12644 ,-13014 , ...
    -13383 ,-13749 ,-14113 ,-14475 ,-14835 , ...
    -15193 ,-15549 ,-15902 ,-16253 ,-16601 , ...
    -16947 ,-17290 ,-17630 ,-17968 ,-18304 , ...
    -18636 ,-18966 ,-19293 ,-19616 ,-19937 , ...
    -20255 ,-20570 ,-20882 ,-21191 ,-21496 , ...
    -21798 ,-22097 ,-22393 ,-22685 ,-22973 , ...
    -23259 ,-23541 ,-23819 ,-24093 ,-24364 , ...
    -24632 ,-24895 ,-25155 ,-25411 ,-25663 , ...
    -25912 ,-26156 ,-26397 ,-26633 ,-26866 , ...
    -27094 ,-27318 ,-27538 ,-27755 ,-27966 , ...
    -28174 ,-28377 ,-28577 ,-28771 ,-28962 , ...
    -29148 ,-29330 ,-29507 ,-29680 ,-29848 , ...
    -30012 ,-30171 ,-30326 ,-30476 ,-30622 , ...
    -30763 ,-30899 ,-31031 ,-31157 ,-31280 , ...
    -31397 ,-31510 ,-31618 ,-31721 ,-31820 , ...
    -31914 ,-32003 ,-32087 ,-32166 ,-32240 , ...
    -32310 ,-32374 ,-32434 ,-32489 ,-32539 , ...
    -32584 ,-32624 ,-32659 ,-32689 ,-32715 , ...
    -32735 ,-32750 ,-32761 ,-32767 ,-32767 , ...
    -32763 ,-32754 ,-32739 ,-32720 ,-32696 , ...
    -32667 ,-32633 ,-32594 ,-32550 ,-32502 , ...
    -32448 ,-32390 ,-32326 ,-32258 ,-32185 , ...
    -32107 ,-32024 ,-31936 ,-31844 ,-31747 , ...
    -31644 ,-31538 ,-31426 ,-31310 ,-31189 , ...
    -31063 ,-30932 ,-30797 ,-30657 ,-30513 , ...
    -30364 ,-30210 ,-30052 ,-29889 ,-29722 , ...
    -29550 ,-29374 ,-29194 ,-29009 ,-28819 , ...
    -28626 ,-28428 ,-28225 ,-28019 ,-27808 , ...
    -27593 ,-27374 ,-27150 ,-26923 ,-26692 , ...
    -26456 ,-26217 ,-25973 ,-25726 ,-25475 , ...
    -25219 ,-24961 ,-24698 ,-24432 ,-24161 , ...
    -23888 ,-23610 ,-23330 ,-23045 ,-22757 , ...
    -22466 ,-22171 ,-21873 ,-21572 ,-21267 , ...
    -20959 ,-20648 ,-20334 ,-20017 ,-19697 , ...
    -19374 ,-19048 ,-18719 ,-18387 ,-18052 , ...
    -17715 ,-17375 ,-17033 ,-16688 ,-16340 , ...
    -15990 ,-15637 ,-15282 ,-14925 ,-14566 , ...
    -14204 ,-13840 ,-13474 ,-13106 ,-12737 , ...
    -12365 ,-11991 ,-11616 ,-11238 ,-10859 , ...
    -10479 ,-10097 , -9713 , -9328 , -8941 , ...
     -8553 , -8164 , -7774 , -7382 , -6989 , ...
     -6596 , -6201 , -5805 , -5409 , -5011 , ...
     -4613 , -4214 , -3815 , -3415 , -3014 , ...
     -2613 , -2212 , -1810 , -1408 , -1006 , ...
      -603 ,  -201 ...
    ]);
end

== matlab function Senorless/FOC_PointModel/MATLAB Function ==
  data: in input; out output; n input
function out = int_shift(in,n)

out = bitshift(in,-n);

== matlab function Senorless/FOC_PointModel/观测器闭环//速度环/PI Controller/积分器/MATLAB Function ==
  data: in input; out output; up input; low input
function out = Limit(in,up,low)

if(in >= up)
    in = up;
end
if(in<= low)
    in = low;
end
out = in;
end

== matlab function Senorless/FOC_PointModel/观测器闭环//速度环/PI Controller/积分器/MATLAB Function1 ==
  data: in input; out output; up input; low input
function out = Limit(in,up,low)

if(in >= up)
    in = up;
end
if(in<= low)
    in = low;
end
out = in;
end

== stateflow chart Senorless/FOC_PointModel/观测器闭环//速度环/NFO速度缓冲 ==
  state Open_Loop
    en:
    du:
    SPD_Ref = SPD_Open;
    ex:
  state SPD_Loop1
    en:
    du:
    SPD_Ref = SPD_MIN;
    ex:
  state SPD_Loop
    en:
    du:
    SPD_Ref = SPD_Loop;
    ex:
  (default) -> Open_Loop
  Open_Loop -> SPD_Loop1 : [after(OPEN_TIME_NFO,sec)]
  SPD_Loop1 -> SPD_Loop : [after(50,msec)]
  data: SPD_Ref output int32; SPD_Open input int32; SPD_Loop input int32; SPD_MIN parameter int32; OPEN_TIME_NFO parameter

== stateflow chart Senorless/FOC_PointModel/观测器闭环//速度环/速度缓冲 ==
  state SPD_Loop
    en:
    du:
    SPD_Ref = SPD_Loop;
    ex:
  state Open_Loop
    en:
    du:
    SPD_Ref = SPD_Open;
    ex:
  (default) -> Open_Loop
  Open_Loop -> SPD_Loop : [after(50,msec)]
  data: SPD_Ref output int32; SPD_Open input int32; SPD_Loop input int32
